simulink model "main_ja"  (R2021b)
settings: Solver=VariableStepAuto  StartTime=0.0  StopTime=10.0  RelTol=1e-3
values from neighbouring files (symbols this model uses):
  d = [dx dy dz]    [init_values.m]
  m = [0.5 0.7 0.5 0.5 0.7]    [TBInertia.m]    (also in init_values.m = 6.33)
  miU_mat_inv = inv([mx*ux' my*uy' mz*uz'])    [init_values.m]
  mx = 0.11    [init_values.m]
  my = 0.11    [init_values.m]
  mz = 0.11    [init_values.m]
  R_o = m_sc * r_off    [init_values.m]
  rhox = [0.1 0 0]    [init_values.m]
  rhoy = [0.1 0 0.1]    [init_values.m]
  rhoz = [0 0 0.1]    [init_values.m]
  ux = [1 0 0]    [init_values.m]
  uy = [0 -1 0]    [init_values.m]
  uz = [0 0 1]    [init_values.m]
libraries: shared6dof x1, simulink x1, vrlib x1
settings Model: Creator=josep  LastModifiedBy=josepfamador

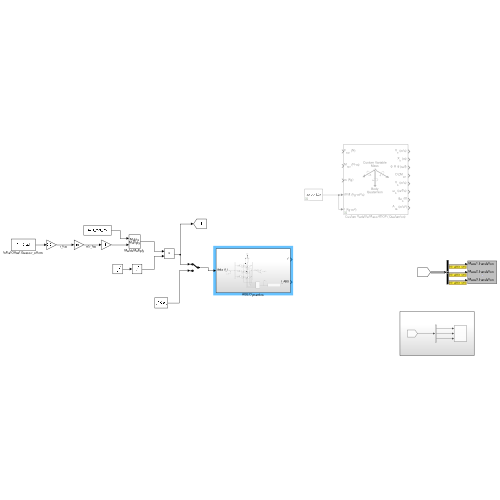
[thumbnail: Simulink's stored preview of the top-level diagram]
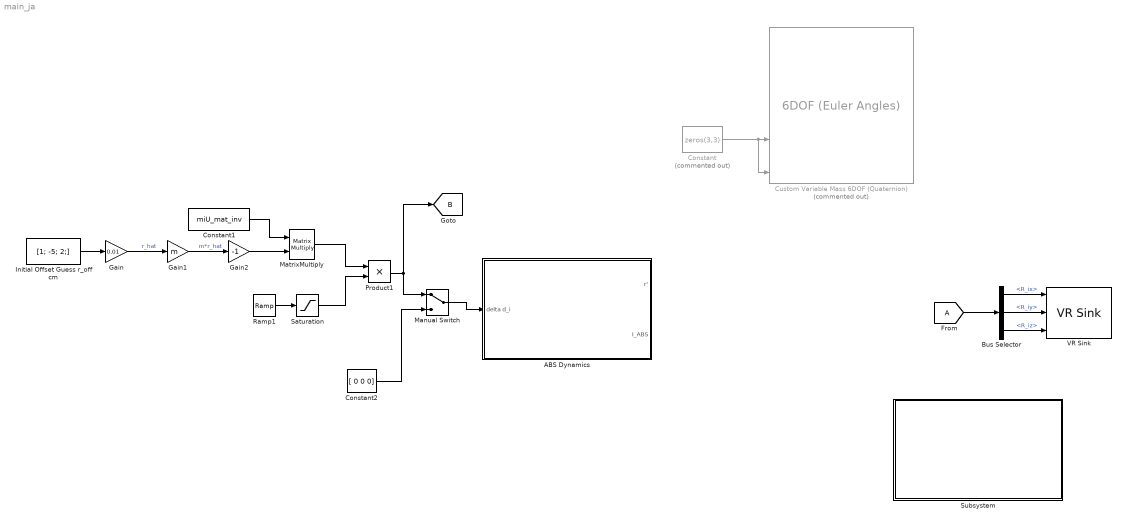
== system main_ja ==
  ABS Dynamics : Subsystem
  Bus Selector : BusSelector  OutputSignals=R_ix,R_iy,R_iz
  Constant : Constant  Commented=on  Value=zeros(3,3)
  Constant1 : Constant  Value=miU_mat_inv
  Constant2 : Constant  Value=[ 0 0 0]
  Custom Variable Mass 6DOF (Quaternion) : shared6dof/6DOF (Euler Angles)  Commented=on  units=Metric (MKS)  mtype=Custom Variable  rep=Quaternion  xme_0=[0 0 0]  Vm_0=[0 0 0]  eul_0=[0 0 0]  pm_0=[0 0 0]  mass_0=1.0  mass_e=0.5  mass_f=2.0  inertia=eye(3)  inertia_e=eye(3)  inertia_f=2*eye(3)  k_quat=1.0  vre_flag=off  abi_flag=off  aMode=0  xme_statename=''  Vm_statename=''  eul_statename=''  quat_statename=''  pm_statename=''  mass_statename=''
      settings: SourceProductBaseCode=AE,PW,DR,MT,UV,VE
  Gain : Gain  Gain=0.01
  Gain1 : Gain  Gain=m
  Gain2 : Gain  Gain=-1
  Initial Offset Guess r_off cm : Constant  Value=[1; -5; 2;]  VectorParams1D=off
  Manual Switch : ManualSwitch
  MatrixMultiply : Product  Multiplication=Matrix(*)
  Product1 : Product
  Ramp1 : simulink/Sources/Ramp  slope=0.1  start=0  InitialOutput=0
  Saturation : Saturate  UpperLimit=1  LowerLimit=0
  Subsystem : Subsystem
  VR Sink : vrlib/VR Sink  InstantiateOnLoad=on  SampleTime=0.1  ViewEnable=on  RemoteChange=off  RemoteView=off  FieldsWritten=Mass1.translation.3.1.1.double#Mass2.translation.3.1.1.double#Mass3.translation.3.1.1.double  WorldFileName=VRSinkFiles/v1.x3d  AutoView=off  VideoDimensions=[]  AllowVariableSize=off
  tag scope: B=global
  wires:
  Constant/1 -> Custom Variable Mass 6DOF (Quaternion)/5, Custom Variable Mass 6DOF (Quaternion)/4
  [A] -> Bus Selector/1
  Bus Selector/1 -> VR Sink/1  "<R_ix>"
  Bus Selector/2 -> VR Sink/2  "<R_iy>"
  Bus Selector/3 -> VR Sink/3  "<R_iz>"
  Product1/1 -> [B], Manual Switch/1
  Constant2/1 -> Manual Switch/2
  Manual Switch/1 -> ABS Dynamics/1(delta d_i)
  Initial Offset Guess r_off cm/1 -> Gain/1
  Gain/1 -> Gain1/1  "r_hat"
  Ramp1/1 -> Saturation/1
  Saturation/1 -> Product1/2
  Gain1/1 -> Gain2/1  "m*r_hat"
  Gain2/1 -> MatrixMultiply/2
  Constant1/1 -> MatrixMultiply/1
  MatrixMultiply/1 -> Product1/1

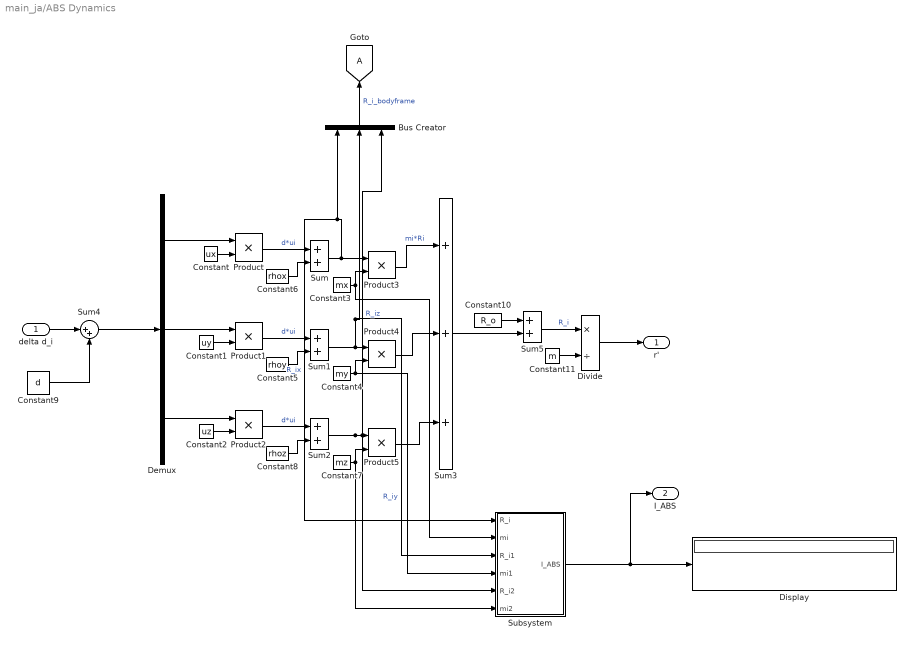
== system main_ja/ABS Dynamics ==
  delta d_i : Inport
  Bus Creator : BusCreator  Inputs=3
  Constant : Constant  Value=ux
  Constant1 : Constant  Value=uy
  Constant10 : Constant  Value=R_o
  Constant11 : Constant  Value=m
  Constant2 : Constant  Value=uz
  Constant3 : Constant  Value=mx
  Constant4 : Constant  Value=my
  Constant5 : Constant  Value=rhoy
  Constant6 : Constant  Value=rhox
  Constant7 : Constant  Value=mz
  Constant8 : Constant  Value=rhoz
  Constant9 : Constant  Value=d
  Demux : Demux  Outputs=3
  Display : Display
  Divide : Product  Inputs=*/
  Product{,1..5} (6 alike) : Product
  Subsystem : Subsystem
  Sum{,1..2,5} (4 alike) : Sum
  Sum3 : Sum  Inputs=+++
  Sum4 : Sum  Inputs=|++
  r' : Outport
  I_ABS : Outport  Port=2
  tag scope: A=global
  wires:
  Demux/1 -> Product/1
  Demux/2 -> Product1/1
  Demux/3 -> Product2/1
  Constant/1 -> Product/2
  Constant1/1 -> Product1/2
  Constant2/1 -> Product2/2
  Product/1 -> Sum/1  "d*ui"
  Constant3/1 -> Product3/2, Subsystem/2(mi)
  Constant6/1 -> Sum/2
  Sum/1 -> Subsystem/1(R_i), Bus Creator/1, Product3/1  "R_ix"
  Sum1/1 -> Bus Creator/2, Subsystem/3(R_i1), Product4/1  "R_iy"
  Constant4/1 -> Product4/2, Subsystem/4(mi1)
  Constant5/1 -> Sum1/2
  Product1/1 -> Sum1/1  "d*ui"
  Sum2/1 -> Bus Creator/3, Subsystem/5(R_i2), Product5/1  "R_iz"
  Constant7/1 -> Subsystem/6(mi2), Product5/2
  Constant8/1 -> Sum2/2
  Product2/1 -> Sum2/1  "d*ui"
  Product3/1 -> Sum3/1  "mi*Ri"
  Product4/1 -> Sum3/2
  Product5/1 -> Sum3/3
  delta d_i/1 -> Sum4/1
  Constant9/1 -> Sum4/2
  Sum4/1 -> Demux/1
  Sum3/1 -> Sum5/2
  Constant10/1 -> Sum5/1
  Sum5/1 -> Divide/1  "R_i"
  Constant11/1 -> Divide/2
  Divide/1 -> r'/1
  Subsystem/1(I_ABS) -> Display/1, I_ABS/1
  Bus Creator/1 -> [A]  "R_i_bodyframe"

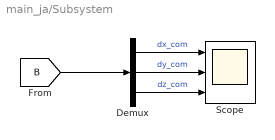
== system main_ja/Subsystem ==
  Demux : Demux  Outputs=3
  Scope : Scope  NumInputPorts=3
  wires:
  [B] -> Demux/1
  Demux/2 -> Scope/2  "dy_com"
  Demux/1 -> Scope/1  "dx_com"
  Demux/3 -> Scope/3  "dz_com"

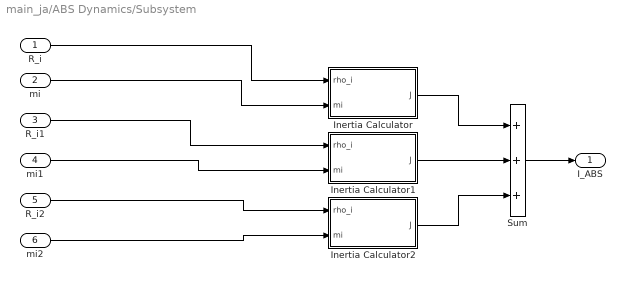
== system main_ja/ABS Dynamics/Subsystem ==
  R_i : Inport
  mi : Inport  Port=2
  R_i1 : Inport  Port=3
  mi1 : Inport  Port=4
  R_i2 : Inport  Port=5
  mi2 : Inport  Port=6
  Inertia Calculator : Subsystem
  Inertia Calculator1 : Subsystem
  Inertia Calculator2 : Subsystem
  Sum : Sum  Inputs=+++
  I_ABS : Outport
  wires:
  mi/1 -> Inertia Calculator/2(mi)
  mi1/1 -> Inertia Calculator1/2(mi)
  R_i/1 -> Inertia Calculator/1(rho_i)
  R_i2/1 -> Inertia Calculator2/1(rho_i)
  R_i1/1 -> Inertia Calculator1/1(rho_i)
  mi2/1 -> Inertia Calculator2/2(mi)
  Inertia Calculator1/1(J) -> Sum/2
  Inertia Calculator/1(J) -> Sum/1
  Inertia Calculator2/1(J) -> Sum/3
  Sum/1 -> I_ABS/1

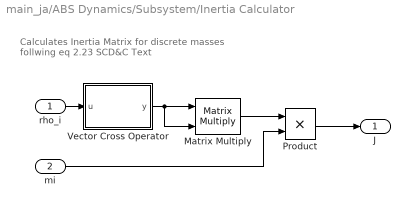
== system main_ja/ABS Dynamics/Subsystem/Inertia Calculator ==
  note: Calculates Inertia Matrix for discrete masses
      | follwing eq 2.23 SCD&C Text
  rho_i : Inport
  mi : Inport  Port=2
  Matrix Multiply : Product  Multiplication=Matrix(*)
  Product : Product
  Vector Cross Operator : MATLAB Function  TreatAsAtomicUnit=on
  J : Outport
  wires:
  Vector Cross Operator/1(y) -> Matrix Multiply/2, Matrix Multiply/1
  rho_i/1 -> Vector Cross Operator/1(u)
  Matrix Multiply/1 -> Product/1
  Product/1 -> J/1
  mi/1 -> Product/2

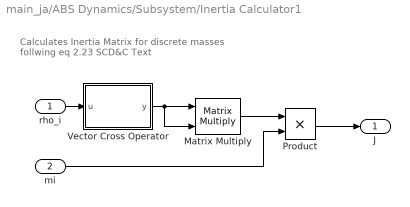
== system main_ja/ABS Dynamics/Subsystem/Inertia Calculator1 ==
  note: Calculates Inertia Matrix for discrete masses
      | follwing eq 2.23 SCD&C Text
  rho_i : Inport
  mi : Inport  Port=2
  Matrix Multiply : Product  Multiplication=Matrix(*)
  Product : Product
  Vector Cross Operator : MATLAB Function  TreatAsAtomicUnit=on
  J : Outport
  wires:
  Vector Cross Operator/1(y) -> Matrix Multiply/2, Matrix Multiply/1
  rho_i/1 -> Vector Cross Operator/1(u)
  Matrix Multiply/1 -> Product/1
  Product/1 -> J/1
  mi/1 -> Product/2

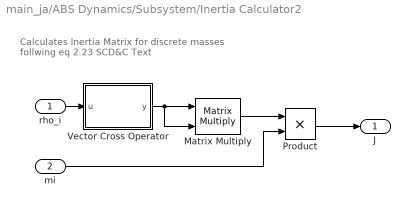
== system main_ja/ABS Dynamics/Subsystem/Inertia Calculator2 ==
  note: Calculates Inertia Matrix for discrete masses
      | follwing eq 2.23 SCD&C Text
  rho_i : Inport
  mi : Inport  Port=2
  Matrix Multiply : Product  Multiplication=Matrix(*)
  Product : Product
  Vector Cross Operator : MATLAB Function  TreatAsAtomicUnit=on
  J : Outport
  wires:
  Vector Cross Operator/1(y) -> Matrix Multiply/2, Matrix Multiply/1
  rho_i/1 -> Vector Cross Operator/1(u)
  Matrix Multiply/1 -> Product/1
  Product/1 -> J/1
  mi/1 -> Product/2

== matlab function main_ja/ABS Dynamics/Subsystem/Inertia Calculator/Vector Cross Operator ==
  data: u input; y output
function y = cross_op(u)
% Rewrites 3x1 vector into Cross product operator
y = [ 0    -u(3)  u(2)
      u(3)  0    -u(1)
     -u(2)  u(1)  0];  %pg 10 S.C. Dyn & Cntrl textbook.

== matlab function main_ja/ABS Dynamics/Subsystem/Inertia Calculator2/Vector Cross Operator ==
  data: u input; y output
function y = cross_op(u)
% Rewrites 3x1 vector into Cross product operator
y = [ 0    -u(3)  u(2)
      u(3)  0    -u(1)
     -u(2)  u(1)  0];  %pg 10 S.C. Dyn & Cntrl textbook.

== matlab function main_ja/ABS Dynamics/Subsystem/Inertia Calculator1/Vector Cross Operator ==
  data: u input; y output
function y = cross_op(u)
% Rewrites 3x1 vector into Cross product operator
y = [ 0    -u(3)  u(2)
      u(3)  0    -u(1)
     -u(2)  u(1)  0];  %pg 10 S.C. Dyn & Cntrl textbook.
